simulink model "simu_unsteady"  (R2020a)
settings: Solver=VariableStepAuto  StartTime=0.0  StopTime=t_final  RelTol=1e-3
values from neighbouring files (symbols this model uses):
  A_lti = - M \ L    [main_unsteady.m]    (also in main_unsteady_validation.m)
  B_lti = M \ [f_omega f_gammaR1 f_gammaQ]    [main_unsteady.m]    (also in main_unsteady_validation.m)
  C_lti = eye(size(A_lti))    [main_unsteady.m]    (also in main_unsteady_validation.m)
  D_lti = zeros(size(B_lti))    [main_unsteady.m]    (also in main_unsteady_validation.m)
  q0 = 0    [main_steadyState.m]    (also in main_steadyState_validation.m; main_unsteady.m; main_unsteady_validation.m)
  reference = 20    [main_unsteady.m]
  T = 20    [main_steadyState.m]    (also in main_steadyState_validation.m = 0; main_unsteady.m = 10; main_unsteady_validation.m = 0)
  T_peak = 3.5    [main_unsteady.m]
  THETA_0 = zeros(n_dof,1) + T    [main_unsteady.m]    (also in main_unsteady_validation.m = (exp(p(nodes_coordinates_full(1,:))) .* exp(g(nodes_coordina)
libraries: cstblocks x1
settings Model: Creator=luigidamico  LastModifiedBy=luigidamico

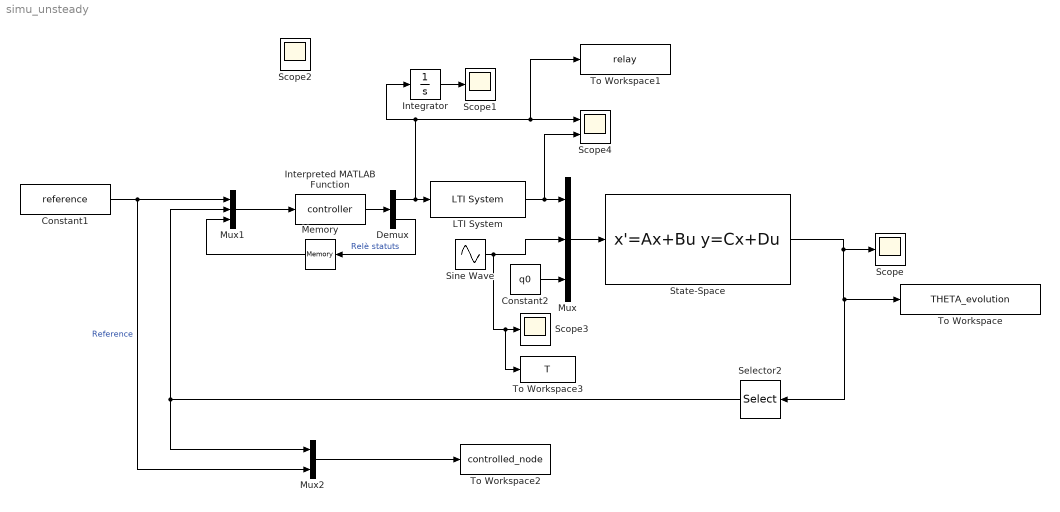
== system simu_unsteady ==
  Constant1 : Constant  Value=reference
  Constant2 : Constant  Value=q0
  Demux : Demux  Outputs=[1 1]
  Integrator : Integrator
  Interpreted MATLAB Function : MATLABFcn  MATLABFcn=controller  OutputDimensions=2  Output1D=off
  LTI System : cstblocks/LTI System  sys=G_s  IC=[]
  Memory : Memory
  Mux : Mux  Inputs=3
  Mux1 : Mux  Inputs=3
  Mux2 : Mux  Inputs=2
  Scope{,1..3} (4 alike) : Scope
  Scope4 : Scope  NumInputPorts=2
  Selector2 : Selector  InputPortWidth=n_dof  IndexOptions=Index vector (dialog)  Indices=idx_sensor  OutputSizes=1
  Sine Wave : Sin  Amplitude=T_peak  Bias=T  Frequency=1/(60*60*24) * 2*pi  Phase=+16/24 * 2*pi  SampleTime=0
  State-Space : StateSpace  A=A_lti  B=B_lti  C=C_lti  D=D_lti  InitialCondition=THETA_0
  To Workspace : ToWorkspace  VariableName=THETA_evolution  SaveFormat=Timeseries  SampleTime=-1
  To Workspace1 : ToWorkspace  VariableName=relay  SaveFormat=Timeseries  SampleTime=-1
  To Workspace2 : ToWorkspace  VariableName=controlled_node  SaveFormat=Timeseries  SampleTime=-1
  To Workspace3 : ToWorkspace  VariableName=T  SaveFormat=Timeseries  SampleTime=-1
  wires:
  Mux/1 -> State-Space/1
  Constant2/1 -> Mux/3
  State-Space/1 -> Scope/1, Selector2/1, To Workspace/1
  Mux1/1 -> Interpreted MATLAB Function/1
  Constant1/1 -> Mux2/2, Mux1/1  "Reference"
  Interpreted MATLAB Function/1 -> Demux/1
  Demux/2 -> Memory/1  "Relè statuts"
  Memory/1 -> Mux1/3
  Demux/1 -> To Workspace1/1, Scope4/1, Integrator/1, LTI System/1
  LTI System/1 -> Mux/1, Scope4/2
  Sine Wave/1 -> To Workspace3/1, Scope3/1, Mux/2
  Selector2/1 -> Mux2/1, Mux1/2
  Mux2/1 -> To Workspace2/1
  Integrator/1 -> Scope1/1
